simulink model "TST_CnvLead_Trq2Q"  (R2016b)
settings: Solver=FixedStepDiscrete  StartTime=0.0  StopTime=simTime  FixedStep=sampleTime  RelTol=1e-3
values from neighbouring files (symbols this model uses):
  testCase = 1    [initTST_CnvLead_Trq2Q_001.m]    (also in initTST_CnvLead_Trq2Q_002.m = 2)
libraries: simulink x9, UnitTest_Lib x6
settings Model: Creator=caijinkang  LastModifiedBy=caijinkang
settings DebuggingCC: SignalRangeChecking=error

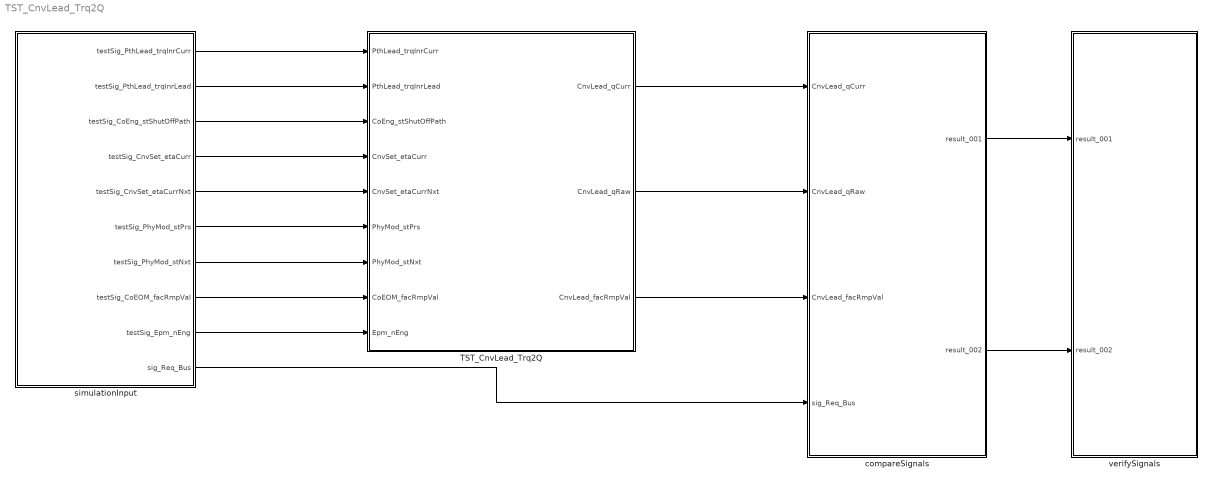
== system TST_CnvLead_Trq2Q ==
  TST_CnvLead_Trq2Q : Subsystem
  compareSignals : Subsystem
  simulationInput : Subsystem
  verifySignals : Subsystem
  wires:
  simulationInput/1(testSig_PthLead_trqInrCurr) -> TST_CnvLead_Trq2Q/1(PthLead_trqInrCurr)
  simulationInput/2(testSig_PthLead_trqInrLead) -> TST_CnvLead_Trq2Q/2(PthLead_trqInrLead)
  simulationInput/3(testSig_CoEng_stShutOffPath) -> TST_CnvLead_Trq2Q/3(CoEng_stShutOffPath)
  simulationInput/4(testSig_CnvSet_etaCurr) -> TST_CnvLead_Trq2Q/4(CnvSet_etaCurr)
  simulationInput/5(testSig_CnvSet_etaCurrNxt) -> TST_CnvLead_Trq2Q/5(CnvSet_etaCurrNxt)
  simulationInput/6(testSig_PhyMod_stPrs) -> TST_CnvLead_Trq2Q/6(PhyMod_stPrs)
  simulationInput/7(testSig_PhyMod_stNxt) -> TST_CnvLead_Trq2Q/7(PhyMod_stNxt)
  simulationInput/8(testSig_CoEOM_facRmpVal) -> TST_CnvLead_Trq2Q/8(CoEOM_facRmpVal)
  simulationInput/9(testSig_Epm_nEng) -> TST_CnvLead_Trq2Q/9(Epm_nEng)
  TST_CnvLead_Trq2Q/1(CnvLead_qCurr) -> compareSignals/1(CnvLead_qCurr)
  TST_CnvLead_Trq2Q/2(CnvLead_qRaw) -> compareSignals/2(CnvLead_qRaw)
  TST_CnvLead_Trq2Q/3(CnvLead_facRmpVal) -> compareSignals/3(CnvLead_facRmpVal)
  simulationInput/10(sig_Req_Bus) -> compareSignals/4(sig_Req_Bus)
  compareSignals/1(result_001) -> verifySignals/1(result_001)
  compareSignals/2(result_002) -> verifySignals/2(result_002)

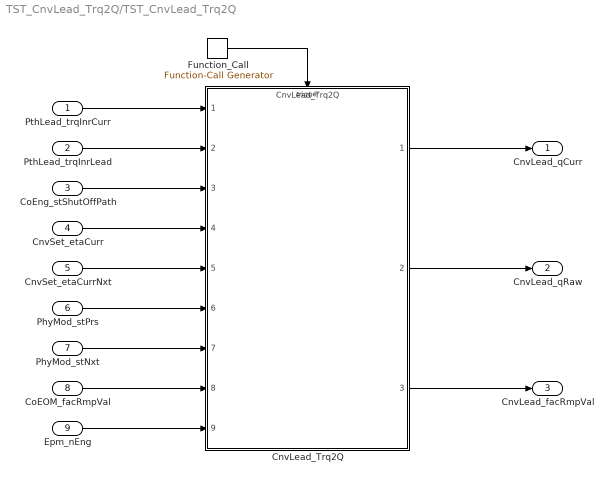
== system TST_CnvLead_Trq2Q/TST_CnvLead_Trq2Q ==
  PthLead_trqInrCurr : Inport
  PthLead_trqInrLead : Inport  Port=2
  CoEng_stShutOffPath : Inport  Port=3
  CnvSet_etaCurr : Inport  Port=4
  CnvSet_etaCurrNxt : Inport  Port=5
  PhyMod_stPrs : Inport  Port=6
  PhyMod_stNxt : Inport  Port=7
  CoEOM_facRmpVal : Inport  Port=8
  Epm_nEng : Inport  Port=9
  CnvLead_Trq2Q : ModelReference  ModelNameDialog=CnvLead_Trq2Q  SimulationMode=Normal  ModelReferenceVersion=1.37  TriggerPortName=function  TriggerPortTriggerType=function-call  TriggerPortStatesWhenEnabling=held
  Function_Call : simulink/Ports & Subsystems/Function-Call Generator  sample_time=sampleTime  numberOfIterations=1
  CnvLead_qCurr : Outport
  CnvLead_qRaw : Outport  Port=2
  CnvLead_facRmpVal : Outport  Port=3
  wires:
  Function_Call/1 -> CnvLead_Trq2Q/Trigger
  PthLead_trqInrCurr/1 -> CnvLead_Trq2Q/1
  PthLead_trqInrLead/1 -> CnvLead_Trq2Q/2
  CoEng_stShutOffPath/1 -> CnvLead_Trq2Q/3
  CnvSet_etaCurr/1 -> CnvLead_Trq2Q/4
  CnvSet_etaCurrNxt/1 -> CnvLead_Trq2Q/5
  PhyMod_stPrs/1 -> CnvLead_Trq2Q/6
  PhyMod_stNxt/1 -> CnvLead_Trq2Q/7
  CoEOM_facRmpVal/1 -> CnvLead_Trq2Q/8
  Epm_nEng/1 -> CnvLead_Trq2Q/9
  CnvLead_Trq2Q/1 -> CnvLead_qCurr/1
  CnvLead_Trq2Q/2 -> CnvLead_qRaw/1
  CnvLead_Trq2Q/3 -> CnvLead_facRmpVal/1

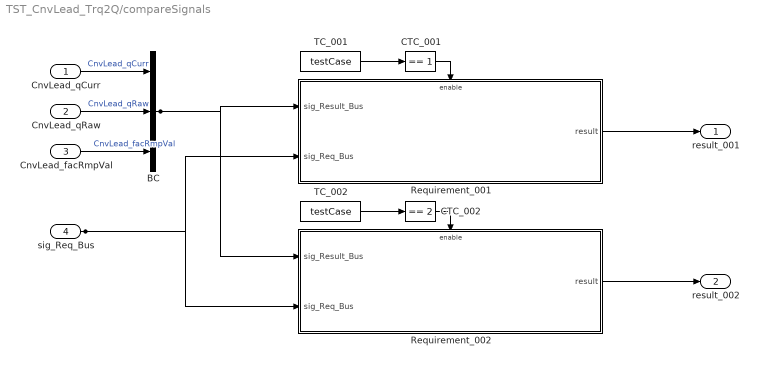
== system TST_CnvLead_Trq2Q/compareSignals ==
  CnvLead_qCurr : Inport
  CnvLead_qRaw : Inport  Port=2
  CnvLead_facRmpVal : Inport  Port=3
  sig_Req_Bus : Inport  Port=4
  BC : BusCreator  Inputs=3
  CTC_001 : simulink/Logic and Bit Operations/Compare To Constant  relop===  const=1  OutDataTypeStr=boolean
  CTC_002 : simulink/Logic and Bit Operations/Compare To Constant  relop===  const=2  OutDataTypeStr=boolean
  Requirement_001 : Subsystem
  Requirement_002 : Subsystem
  TC_001 : Constant  Value=testCase
  TC_002 : Constant  Value=testCase
  result_001 : Outport
  result_002 : Outport  Port=2
  wires:
  CnvLead_qCurr/1 -> BC/1  "CnvLead_qCurr"
  CnvLead_qRaw/1 -> BC/2  "CnvLead_qRaw"
  CnvLead_facRmpVal/1 -> BC/3  "CnvLead_facRmpVal"
  TC_001/1 -> CTC_001/1
  CTC_001/1 -> Requirement_001/Enable
  sig_Req_Bus/1 -> Requirement_001/2(sig_Req_Bus), Requirement_002/2(sig_Req_Bus)
  BC/1 -> Requirement_001/1(sig_Result_Bus), Requirement_002/1(sig_Result_Bus)
  Requirement_001/1(result) -> result_001/1
  TC_002/1 -> CTC_002/1
  CTC_002/1 -> Requirement_002/Enable
  Requirement_002/1(result) -> result_002/1

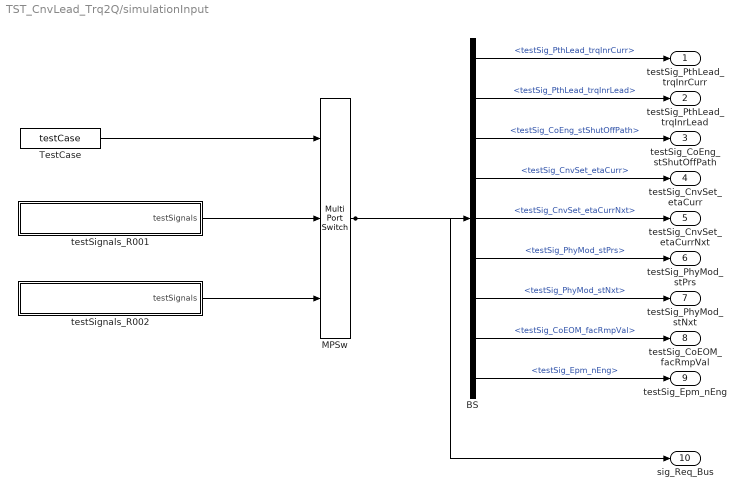
== system TST_CnvLead_Trq2Q/simulationInput ==
  BS : BusSelector  OutputSignals=testSig_PthLead_trqInrCurr,testSig_PthLead_trqInrLead,testSig_CoEng_stShutOffPath,testSig_CnvSet_etaCurr,testSig_CnvSet_etaCurrNxt,testSig_PhyMod_stPrs,testSig_PhyMod_stNxt,testSig_CoEOM_facRmpVal,testSig_Epm_nEng
  MPSw : MultiPortSwitch  Inputs=2  SaturateOnIntegerOverflow=on  InputSameDT=on
  TestCase : Constant  Value=testCase
  testSignals_R001 : Subsystem
  testSignals_R002 : Subsystem
  testSig_PthLead_trqInrCurr : Outport
  testSig_PthLead_trqInrLead : Outport  Port=2
  testSig_CoEng_stShutOffPath : Outport  Port=3
  testSig_CnvSet_etaCurr : Outport  Port=4
  testSig_CnvSet_etaCurrNxt : Outport  Port=5
  testSig_PhyMod_stPrs : Outport  Port=6
  testSig_PhyMod_stNxt : Outport  Port=7
  testSig_CoEOM_facRmpVal : Outport  Port=8
  testSig_Epm_nEng : Outport  Port=9
  sig_Req_Bus : Outport  Port=10
  wires:
  BS/1 -> testSig_PthLead_trqInrCurr/1  "<testSig_PthLead_trqInrCurr>"
  BS/2 -> testSig_PthLead_trqInrLead/1  "<testSig_PthLead_trqInrLead>"
  BS/3 -> testSig_CoEng_stShutOffPath/1  "<testSig_CoEng_stShutOffPath>"
  BS/4 -> testSig_CnvSet_etaCurr/1  "<testSig_CnvSet_etaCurr>"
  BS/5 -> testSig_CnvSet_etaCurrNxt/1  "<testSig_CnvSet_etaCurrNxt>"
  BS/6 -> testSig_PhyMod_stPrs/1  "<testSig_PhyMod_stPrs>"
  BS/7 -> testSig_PhyMod_stNxt/1  "<testSig_PhyMod_stNxt>"
  BS/8 -> testSig_CoEOM_facRmpVal/1  "<testSig_CoEOM_facRmpVal>"
  BS/9 -> testSig_Epm_nEng/1  "<testSig_Epm_nEng>"
  MPSw/1 -> BS/1, sig_Req_Bus/1
  TestCase/1 -> MPSw/1
  testSignals_R001/1(testSignals) -> MPSw/2
  testSignals_R002/1(testSignals) -> MPSw/3

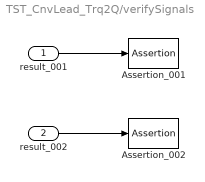
== system TST_CnvLead_Trq2Q/verifySignals ==
  result_001 : Inport
  result_002 : Inport  Port=2
  Assertion_001 : Assertion  Enabled=off
  Assertion_002 : Assertion  Enabled=off
  wires:
  result_001/1 -> Assertion_001/1
  result_002/1 -> Assertion_002/1

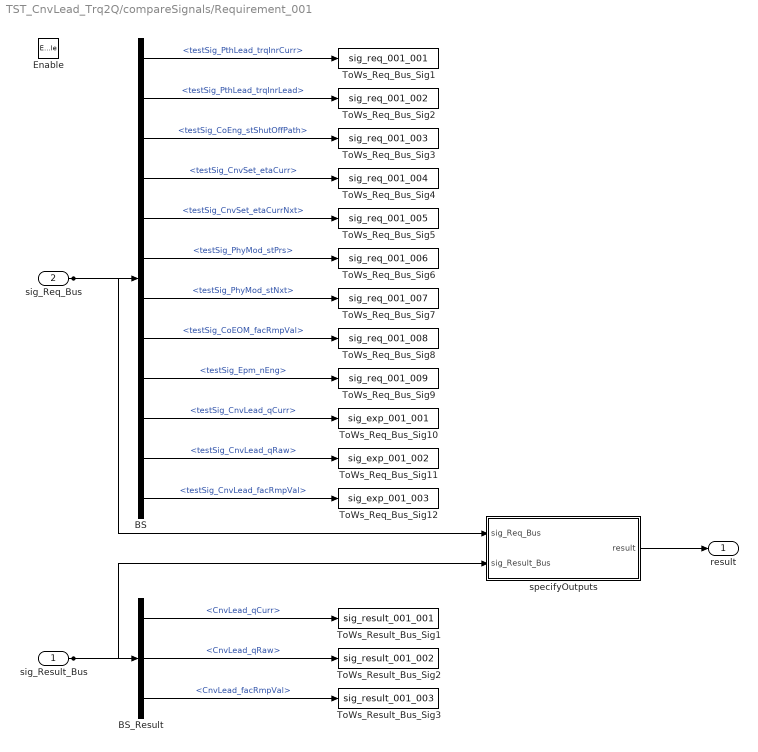
== system TST_CnvLead_Trq2Q/compareSignals/Requirement_001 ==
  sig_Result_Bus : Inport
  sig_Req_Bus : Inport  Port=2
  Enable : EnablePort
  BS : BusSelector  OutputSignals=testSig_PthLead_trqInrCurr,testSig_PthLead_trqInrLead,testSig_CoEng_stShutOffPath,testSig_CnvSet_etaCurr,testSig_CnvSet_etaCurrNxt,testSig_PhyMod_stPrs,testSig_PhyMod_stNxt,testSig_CoEOM_facRmpVal,testSig_Epm_nEng,testSig_CnvLead_qCurr,testSig_CnvLead_qRaw,testSig_CnvLead_facRmpVal
  BS_Result : BusSelector  OutputSignals=CnvLead_qCurr,CnvLead_qRaw,CnvLead_facRmpVal
  ToWs_Req_Bus_Sig1 : ToWorkspace  VariableName=sig_req_001_001  SaveFormat=Structure With Time
  ToWs_Req_Bus_Sig10 : ToWorkspace  VariableName=sig_exp_001_001  SaveFormat=Structure With Time
  ToWs_Req_Bus_Sig11 : ToWorkspace  VariableName=sig_exp_001_002  SaveFormat=Structure With Time
  ToWs_Req_Bus_Sig12 : ToWorkspace  VariableName=sig_exp_001_003  SaveFormat=Structure With Time
  ToWs_Req_Bus_Sig2 : ToWorkspace  VariableName=sig_req_001_002  SaveFormat=Structure With Time
  ToWs_Req_Bus_Sig3 : ToWorkspace  VariableName=sig_req_001_003  SaveFormat=Structure With Time
  ToWs_Req_Bus_Sig4 : ToWorkspace  VariableName=sig_req_001_004  SaveFormat=Structure With Time
  ToWs_Req_Bus_Sig5 : ToWorkspace  VariableName=sig_req_001_005  SaveFormat=Structure With Time
  ToWs_Req_Bus_Sig6 : ToWorkspace  VariableName=sig_req_001_006  SaveFormat=Structure With Time
  ToWs_Req_Bus_Sig7 : ToWorkspace  VariableName=sig_req_001_007  SaveFormat=Structure With Time
  ToWs_Req_Bus_Sig8 : ToWorkspace  VariableName=sig_req_001_008  SaveFormat=Structure With Time
  ToWs_Req_Bus_Sig9 : ToWorkspace  VariableName=sig_req_001_009  SaveFormat=Structure With Time
  ToWs_Result_Bus_Sig1 : ToWorkspace  VariableName=sig_result_001_001  SaveFormat=Structure With Time
  ToWs_Result_Bus_Sig2 : ToWorkspace  VariableName=sig_result_001_002  SaveFormat=Structure With Time
  ToWs_Result_Bus_Sig3 : ToWorkspace  VariableName=sig_result_001_003  SaveFormat=Structure With Time
  specifyOutputs : Subsystem
  result : Outport
  wires:
  sig_Req_Bus/1 -> BS/1, specifyOutputs/1(sig_Req_Bus)
  BS/1 -> ToWs_Req_Bus_Sig1/1  "<testSig_PthLead_trqInrCurr>"
  BS/2 -> ToWs_Req_Bus_Sig2/1  "<testSig_PthLead_trqInrLead>"
  BS/3 -> ToWs_Req_Bus_Sig3/1  "<testSig_CoEng_stShutOffPath>"
  BS/4 -> ToWs_Req_Bus_Sig4/1  "<testSig_CnvSet_etaCurr>"
  BS/5 -> ToWs_Req_Bus_Sig5/1  "<testSig_CnvSet_etaCurrNxt>"
  BS/6 -> ToWs_Req_Bus_Sig6/1  "<testSig_PhyMod_stPrs>"
  BS/7 -> ToWs_Req_Bus_Sig7/1  "<testSig_PhyMod_stNxt>"
  BS/8 -> ToWs_Req_Bus_Sig8/1  "<testSig_CoEOM_facRmpVal>"
  BS/9 -> ToWs_Req_Bus_Sig9/1  "<testSig_Epm_nEng>"
  BS/10 -> ToWs_Req_Bus_Sig10/1  "<testSig_CnvLead_qCurr>"
  BS/11 -> ToWs_Req_Bus_Sig11/1  "<testSig_CnvLead_qRaw>"
  BS/12 -> ToWs_Req_Bus_Sig12/1  "<testSig_CnvLead_facRmpVal>"
  sig_Result_Bus/1 -> BS_Result/1, specifyOutputs/2(sig_Result_Bus)
  BS_Result/1 -> ToWs_Result_Bus_Sig1/1  "<CnvLead_qCurr>"
  BS_Result/2 -> ToWs_Result_Bus_Sig2/1  "<CnvLead_qRaw>"
  BS_Result/3 -> ToWs_Result_Bus_Sig3/1  "<CnvLead_facRmpVal>"
  specifyOutputs/1(result) -> result/1

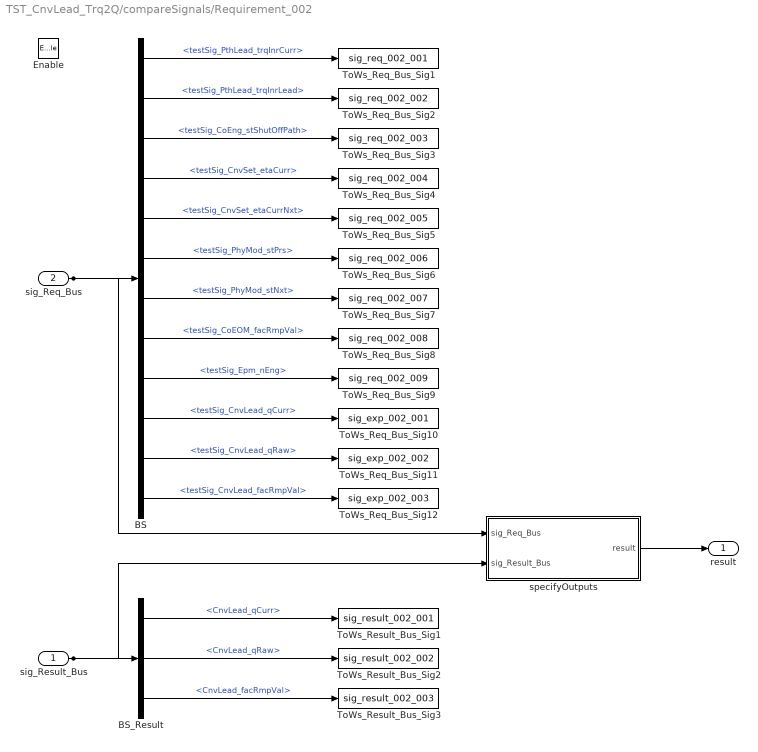
== system TST_CnvLead_Trq2Q/compareSignals/Requirement_002 ==
  sig_Result_Bus : Inport
  sig_Req_Bus : Inport  Port=2
  Enable : EnablePort
  BS : BusSelector  OutputSignals=testSig_PthLead_trqInrCurr,testSig_PthLead_trqInrLead,testSig_CoEng_stShutOffPath,testSig_CnvSet_etaCurr,testSig_CnvSet_etaCurrNxt,testSig_PhyMod_stPrs,testSig_PhyMod_stNxt,testSig_CoEOM_facRmpVal,testSig_Epm_nEng,testSig_CnvLead_qCurr,testSig_CnvLead_qRaw,testSig_CnvLead_facRmpVal
  BS_Result : BusSelector  OutputSignals=CnvLead_qCurr,CnvLead_qRaw,CnvLead_facRmpVal
  ToWs_Req_Bus_Sig1 : ToWorkspace  VariableName=sig_req_002_001  SaveFormat=Structure With Time
  ToWs_Req_Bus_Sig10 : ToWorkspace  VariableName=sig_exp_002_001  SaveFormat=Structure With Time
  ToWs_Req_Bus_Sig11 : ToWorkspace  VariableName=sig_exp_002_002  SaveFormat=Structure With Time
  ToWs_Req_Bus_Sig12 : ToWorkspace  VariableName=sig_exp_002_003  SaveFormat=Structure With Time
  ToWs_Req_Bus_Sig2 : ToWorkspace  VariableName=sig_req_002_002  SaveFormat=Structure With Time
  ToWs_Req_Bus_Sig3 : ToWorkspace  VariableName=sig_req_002_003  SaveFormat=Structure With Time
  ToWs_Req_Bus_Sig4 : ToWorkspace  VariableName=sig_req_002_004  SaveFormat=Structure With Time
  ToWs_Req_Bus_Sig5 : ToWorkspace  VariableName=sig_req_002_005  SaveFormat=Structure With Time
  ToWs_Req_Bus_Sig6 : ToWorkspace  VariableName=sig_req_002_006  SaveFormat=Structure With Time
  ToWs_Req_Bus_Sig7 : ToWorkspace  VariableName=sig_req_002_007  SaveFormat=Structure With Time
  ToWs_Req_Bus_Sig8 : ToWorkspace  VariableName=sig_req_002_008  SaveFormat=Structure With Time
  ToWs_Req_Bus_Sig9 : ToWorkspace  VariableName=sig_req_002_009  SaveFormat=Structure With Time
  ToWs_Result_Bus_Sig1 : ToWorkspace  VariableName=sig_result_002_001  SaveFormat=Structure With Time
  ToWs_Result_Bus_Sig2 : ToWorkspace  VariableName=sig_result_002_002  SaveFormat=Structure With Time
  ToWs_Result_Bus_Sig3 : ToWorkspace  VariableName=sig_result_002_003  SaveFormat=Structure With Time
  specifyOutputs : Subsystem
  result : Outport
  wires:
  sig_Req_Bus/1 -> BS/1, specifyOutputs/1(sig_Req_Bus)
  BS/1 -> ToWs_Req_Bus_Sig1/1  "<testSig_PthLead_trqInrCurr>"
  BS/2 -> ToWs_Req_Bus_Sig2/1  "<testSig_PthLead_trqInrLead>"
  BS/3 -> ToWs_Req_Bus_Sig3/1  "<testSig_CoEng_stShutOffPath>"
  BS/4 -> ToWs_Req_Bus_Sig4/1  "<testSig_CnvSet_etaCurr>"
  BS/5 -> ToWs_Req_Bus_Sig5/1  "<testSig_CnvSet_etaCurrNxt>"
  BS/6 -> ToWs_Req_Bus_Sig6/1  "<testSig_PhyMod_stPrs>"
  BS/7 -> ToWs_Req_Bus_Sig7/1  "<testSig_PhyMod_stNxt>"
  BS/8 -> ToWs_Req_Bus_Sig8/1  "<testSig_CoEOM_facRmpVal>"
  BS/9 -> ToWs_Req_Bus_Sig9/1  "<testSig_Epm_nEng>"
  BS/10 -> ToWs_Req_Bus_Sig10/1  "<testSig_CnvLead_qCurr>"
  BS/11 -> ToWs_Req_Bus_Sig11/1  "<testSig_CnvLead_qRaw>"
  BS/12 -> ToWs_Req_Bus_Sig12/1  "<testSig_CnvLead_facRmpVal>"
  sig_Result_Bus/1 -> BS_Result/1, specifyOutputs/2(sig_Result_Bus)
  BS_Result/1 -> ToWs_Result_Bus_Sig1/1  "<CnvLead_qCurr>"
  BS_Result/2 -> ToWs_Result_Bus_Sig2/1  "<CnvLead_qRaw>"
  BS_Result/3 -> ToWs_Result_Bus_Sig3/1  "<CnvLead_facRmpVal>"
  specifyOutputs/1(result) -> result/1

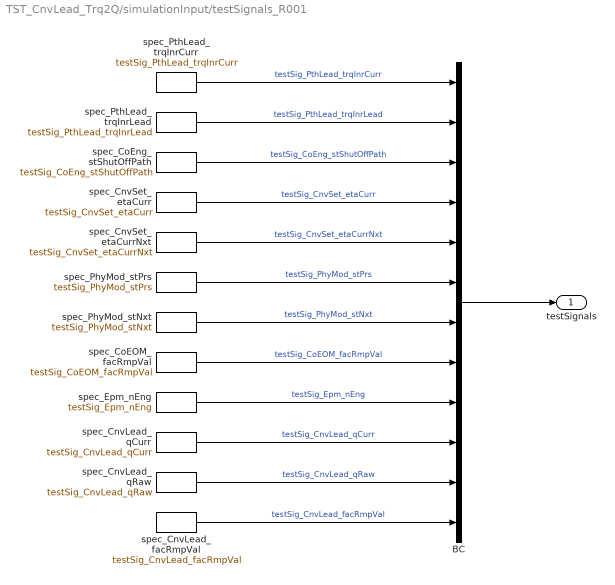
== system TST_CnvLead_Trq2Q/simulationInput/testSignals_R001 ==
  BC : BusCreator  Inputs=12
  spec_CnvLead_facRmpVal : FromWorkspace  VariableName=testSig_CnvLead_facRmpVal  Interpolate=off  OutputAfterFinalValue=Holding final value
  spec_CnvLead_qCurr : FromWorkspace  VariableName=testSig_CnvLead_qCurr  Interpolate=off  OutputAfterFinalValue=Holding final value
  spec_CnvLead_qRaw : FromWorkspace  VariableName=testSig_CnvLead_qRaw  Interpolate=off  OutputAfterFinalValue=Holding final value
  spec_CnvSet_etaCurr : FromWorkspace  VariableName=testSig_CnvSet_etaCurr  Interpolate=off  OutputAfterFinalValue=Holding final value
  spec_CnvSet_etaCurrNxt : FromWorkspace  VariableName=testSig_CnvSet_etaCurrNxt  Interpolate=off  OutputAfterFinalValue=Holding final value
  spec_CoEOM_facRmpVal : FromWorkspace  VariableName=testSig_CoEOM_facRmpVal  Interpolate=off  OutputAfterFinalValue=Holding final value
  spec_CoEng_stShutOffPath : FromWorkspace  VariableName=testSig_CoEng_stShutOffPath  Interpolate=off  OutputAfterFinalValue=Holding final value
  spec_Epm_nEng : FromWorkspace  VariableName=testSig_Epm_nEng  Interpolate=off  OutputAfterFinalValue=Holding final value
  spec_PhyMod_stNxt : FromWorkspace  VariableName=testSig_PhyMod_stNxt  Interpolate=off  OutputAfterFinalValue=Holding final value
  spec_PhyMod_stPrs : FromWorkspace  VariableName=testSig_PhyMod_stPrs  Interpolate=off  OutputAfterFinalValue=Holding final value
  spec_PthLead_trqInrCurr : FromWorkspace  VariableName=testSig_PthLead_trqInrCurr  Interpolate=off  OutputAfterFinalValue=Holding final value
  spec_PthLead_trqInrLead : FromWorkspace  VariableName=testSig_PthLead_trqInrLead  Interpolate=off  OutputAfterFinalValue=Holding final value
  testSignals : Outport
  wires:
  BC/1 -> testSignals/1
  spec_PthLead_trqInrCurr/1 -> BC/1  "testSig_PthLead_trqInrCurr"
  spec_PthLead_trqInrLead/1 -> BC/2  "testSig_PthLead_trqInrLead"
  spec_CoEng_stShutOffPath/1 -> BC/3  "testSig_CoEng_stShutOffPath"
  spec_CnvSet_etaCurr/1 -> BC/4  "testSig_CnvSet_etaCurr"
  spec_CnvSet_etaCurrNxt/1 -> BC/5  "testSig_CnvSet_etaCurrNxt"
  spec_PhyMod_stPrs/1 -> BC/6  "testSig_PhyMod_stPrs"
  spec_PhyMod_stNxt/1 -> BC/7  "testSig_PhyMod_stNxt"
  spec_CoEOM_facRmpVal/1 -> BC/8  "testSig_CoEOM_facRmpVal"
  spec_Epm_nEng/1 -> BC/9  "testSig_Epm_nEng"
  spec_CnvLead_qCurr/1 -> BC/10  "testSig_CnvLead_qCurr"
  spec_CnvLead_qRaw/1 -> BC/11  "testSig_CnvLead_qRaw"
  spec_CnvLead_facRmpVal/1 -> BC/12  "testSig_CnvLead_facRmpVal"

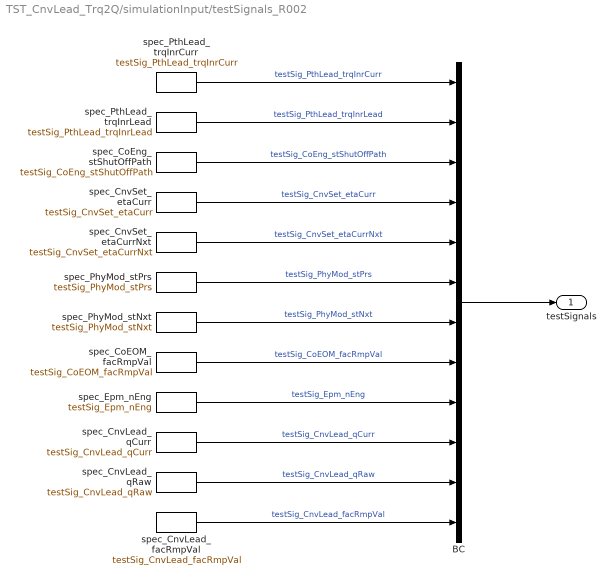
== system TST_CnvLead_Trq2Q/simulationInput/testSignals_R002 ==
  BC : BusCreator  Inputs=12
  spec_CnvLead_facRmpVal : FromWorkspace  VariableName=testSig_CnvLead_facRmpVal  Interpolate=off  OutputAfterFinalValue=Holding final value
  spec_CnvLead_qCurr : FromWorkspace  VariableName=testSig_CnvLead_qCurr  Interpolate=off  OutputAfterFinalValue=Holding final value
  spec_CnvLead_qRaw : FromWorkspace  VariableName=testSig_CnvLead_qRaw  Interpolate=off  OutputAfterFinalValue=Holding final value
  spec_CnvSet_etaCurr : FromWorkspace  VariableName=testSig_CnvSet_etaCurr  Interpolate=off  OutputAfterFinalValue=Holding final value
  spec_CnvSet_etaCurrNxt : FromWorkspace  VariableName=testSig_CnvSet_etaCurrNxt  Interpolate=off  OutputAfterFinalValue=Holding final value
  spec_CoEOM_facRmpVal : FromWorkspace  VariableName=testSig_CoEOM_facRmpVal  Interpolate=off  OutputAfterFinalValue=Holding final value
  spec_CoEng_stShutOffPath : FromWorkspace  VariableName=testSig_CoEng_stShutOffPath  Interpolate=off  OutputAfterFinalValue=Holding final value
  spec_Epm_nEng : FromWorkspace  VariableName=testSig_Epm_nEng  Interpolate=off  OutputAfterFinalValue=Holding final value
  spec_PhyMod_stNxt : FromWorkspace  VariableName=testSig_PhyMod_stNxt  Interpolate=off  OutputAfterFinalValue=Holding final value
  spec_PhyMod_stPrs : FromWorkspace  VariableName=testSig_PhyMod_stPrs  Interpolate=off  OutputAfterFinalValue=Holding final value
  spec_PthLead_trqInrCurr : FromWorkspace  VariableName=testSig_PthLead_trqInrCurr  Interpolate=off  OutputAfterFinalValue=Holding final value
  spec_PthLead_trqInrLead : FromWorkspace  VariableName=testSig_PthLead_trqInrLead  Interpolate=off  OutputAfterFinalValue=Holding final value
  testSignals : Outport
  wires:
  BC/1 -> testSignals/1
  spec_PthLead_trqInrCurr/1 -> BC/1  "testSig_PthLead_trqInrCurr"
  spec_PthLead_trqInrLead/1 -> BC/2  "testSig_PthLead_trqInrLead"
  spec_CoEng_stShutOffPath/1 -> BC/3  "testSig_CoEng_stShutOffPath"
  spec_CnvSet_etaCurr/1 -> BC/4  "testSig_CnvSet_etaCurr"
  spec_CnvSet_etaCurrNxt/1 -> BC/5  "testSig_CnvSet_etaCurrNxt"
  spec_PhyMod_stPrs/1 -> BC/6  "testSig_PhyMod_stPrs"
  spec_PhyMod_stNxt/1 -> BC/7  "testSig_PhyMod_stNxt"
  spec_CoEOM_facRmpVal/1 -> BC/8  "testSig_CoEOM_facRmpVal"
  spec_Epm_nEng/1 -> BC/9  "testSig_Epm_nEng"
  spec_CnvLead_qCurr/1 -> BC/10  "testSig_CnvLead_qCurr"
  spec_CnvLead_qRaw/1 -> BC/11  "testSig_CnvLead_qRaw"
  spec_CnvLead_facRmpVal/1 -> BC/12  "testSig_CnvLead_facRmpVal"

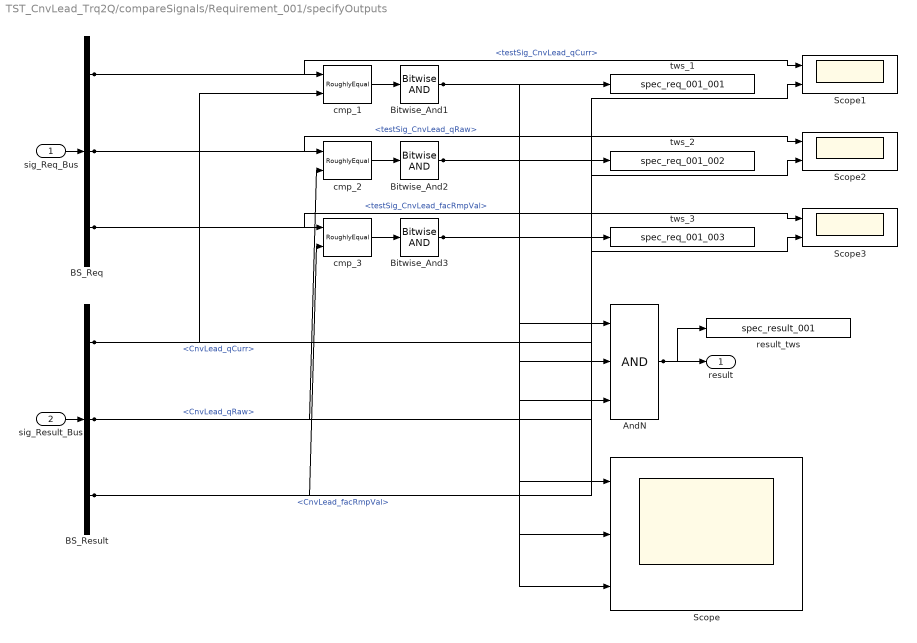
== system TST_CnvLead_Trq2Q/compareSignals/Requirement_001/specifyOutputs ==
  sig_Req_Bus : Inport
  sig_Result_Bus : Inport  Port=2
  AndN : Logic  Inputs=3
  BS_Req : BusSelector  OutputSignals=testSig_CnvLead_qCurr,testSig_CnvLead_qRaw,testSig_CnvLead_facRmpVal
  BS_Result : BusSelector  OutputSignals=CnvLead_qCurr,CnvLead_qRaw,CnvLead_facRmpVal
  Bitwise_And1 : simulink/Logic and Bit Operations/Bitwise Operator  logicop=AND  UseBitMask=off  BitMask=bin2dec('11011001')  BitMaskRealWorld=Stored Integer
  Bitwise_And2 : simulink/Logic and Bit Operations/Bitwise Operator  logicop=AND  UseBitMask=off  BitMask=bin2dec('11011001')  BitMaskRealWorld=Stored Integer
  Bitwise_And3 : simulink/Logic and Bit Operations/Bitwise Operator  logicop=AND  UseBitMask=off  BitMask=bin2dec('11011001')  BitMaskRealWorld=Stored Integer
  Scope : Scope  NumInputPorts=3
  Scope1 : Scope  NumInputPorts=2
  Scope2 : Scope  NumInputPorts=2
  Scope3 : Scope  NumInputPorts=2
  cmp_1 : UnitTest_Lib/RoughlyEqual  slope=0.1
  cmp_2 : UnitTest_Lib/RoughlyEqual  slope=0.1
  cmp_3 : UnitTest_Lib/RoughlyEqual  slope=0.1
  result_tws : ToWorkspace  VariableName=spec_result_001
  tws_1 : ToWorkspace  VariableName=spec_req_001_001
  tws_2 : ToWorkspace  VariableName=spec_req_001_002
  tws_3 : ToWorkspace  VariableName=spec_req_001_003
  result : Outport
  wires:
  sig_Req_Bus/1 -> BS_Req/1
  sig_Result_Bus/1 -> BS_Result/1
  AndN/1 -> result/1, result_tws/1
  BS_Req/1 -> cmp_1/1, Scope1/1  "<testSig_CnvLead_qCurr>"
  BS_Result/1 -> cmp_1/2, Scope1/2  "<CnvLead_qCurr>"
  cmp_1/1 -> Bitwise_And1/1
  Bitwise_And1/1 -> tws_1/1, AndN/1, Scope/1
  BS_Req/2 -> cmp_2/1, Scope2/1  "<testSig_CnvLead_qRaw>"
  BS_Result/2 -> cmp_2/2, Scope2/2  "<CnvLead_qRaw>"
  cmp_2/1 -> Bitwise_And2/1
  Bitwise_And2/1 -> tws_2/1, AndN/2, Scope/2
  BS_Req/3 -> cmp_3/1, Scope3/1  "<testSig_CnvLead_facRmpVal>"
  BS_Result/3 -> cmp_3/2, Scope3/2  "<CnvLead_facRmpVal>"
  cmp_3/1 -> Bitwise_And3/1
  Bitwise_And3/1 -> tws_3/1, AndN/3, Scope/3

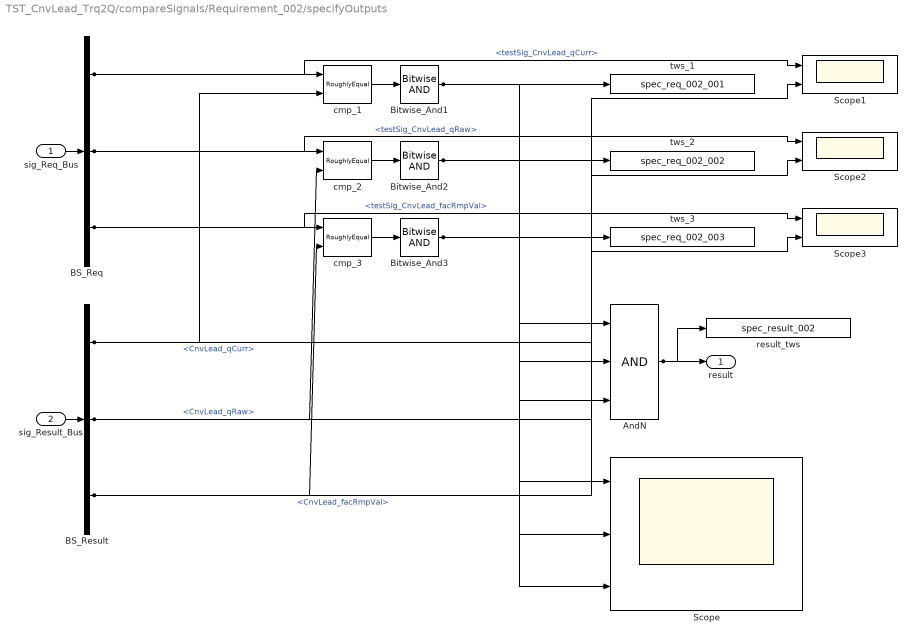
== system TST_CnvLead_Trq2Q/compareSignals/Requirement_002/specifyOutputs ==
  sig_Req_Bus : Inport
  sig_Result_Bus : Inport  Port=2
  AndN : Logic  Inputs=3
  BS_Req : BusSelector  OutputSignals=testSig_CnvLead_qCurr,testSig_CnvLead_qRaw,testSig_CnvLead_facRmpVal
  BS_Result : BusSelector  OutputSignals=CnvLead_qCurr,CnvLead_qRaw,CnvLead_facRmpVal
  Bitwise_And1 : simulink/Logic and Bit Operations/Bitwise Operator  logicop=AND  UseBitMask=off  BitMask=bin2dec('11011001')  BitMaskRealWorld=Stored Integer
  Bitwise_And2 : simulink/Logic and Bit Operations/Bitwise Operator  logicop=AND  UseBitMask=off  BitMask=bin2dec('11011001')  BitMaskRealWorld=Stored Integer
  Bitwise_And3 : simulink/Logic and Bit Operations/Bitwise Operator  logicop=AND  UseBitMask=off  BitMask=bin2dec('11011001')  BitMaskRealWorld=Stored Integer
  Scope : Scope  NumInputPorts=3
  Scope1 : Scope  NumInputPorts=2
  Scope2 : Scope  NumInputPorts=2
  Scope3 : Scope  NumInputPorts=2
  cmp_1 : UnitTest_Lib/RoughlyEqual  slope=0.1
  cmp_2 : UnitTest_Lib/RoughlyEqual  slope=0.1
  cmp_3 : UnitTest_Lib/RoughlyEqual  slope=0.1
  result_tws : ToWorkspace  VariableName=spec_result_002
  tws_1 : ToWorkspace  VariableName=spec_req_002_001
  tws_2 : ToWorkspace  VariableName=spec_req_002_002
  tws_3 : ToWorkspace  VariableName=spec_req_002_003
  result : Outport
  wires:
  sig_Req_Bus/1 -> BS_Req/1
  sig_Result_Bus/1 -> BS_Result/1
  AndN/1 -> result/1, result_tws/1
  BS_Req/1 -> cmp_1/1, Scope1/1  "<testSig_CnvLead_qCurr>"
  BS_Result/1 -> cmp_1/2, Scope1/2  "<CnvLead_qCurr>"
  cmp_1/1 -> Bitwise_And1/1
  Bitwise_And1/1 -> tws_1/1, AndN/1, Scope/1
  BS_Req/2 -> cmp_2/1, Scope2/1  "<testSig_CnvLead_qRaw>"
  BS_Result/2 -> cmp_2/2, Scope2/2  "<CnvLead_qRaw>"
  cmp_2/1 -> Bitwise_And2/1
  Bitwise_And2/1 -> tws_2/1, AndN/2, Scope/2
  BS_Req/3 -> cmp_3/1, Scope3/1  "<testSig_CnvLead_facRmpVal>"
  BS_Result/3 -> cmp_3/2, Scope3/2  "<CnvLead_facRmpVal>"
  cmp_3/1 -> Bitwise_And3/1
  Bitwise_And3/1 -> tws_3/1, AndN/3, Scope/3
